simulink model "computer_detect_trafficlight"  (R2016b)
settings: Solver=VariableStepAuto  StartTime=0.0  StopTime=inf  RelTol=1e-3
values from neighbouring files (symbols this model uses):
  h_max_r = hmax(size(hmax,2))    [com_getColor_red.m]    (also in computer_getColor_red.m; computer_getColor_red_video.m)
  h_min_r = hmin(size(hmin,2))    [com_getColor_red.m]    (also in computer_getColor_red.m; computer_getColor_red_video.m)
  s_max_r = smax(size(smax,2))    [com_getColor_red.m]    (also in computer_getColor_red.m; computer_getColor_red_video.m)
  s_min_r = smin(size(smin,2))    [com_getColor_red.m]    (also in computer_getColor_red.m; computer_getColor_red_video.m)
  v_max_r = vmax(size(vmax,2))    [com_getColor_red.m]    (also in computer_getColor_red.m; computer_getColor_red_video.m)
  v_min_r = vmin(size(vmin,2))    [com_getColor_red.m]    (also in computer_getColor_red.m; computer_getColor_red_video.m)
undefined symbols (not defined in the file or in its folder): gray, Rec, SDTV, strel
libraries: dspnetwork x15, visionconversions x5, visionmorphops x2, visiontextngfix x1, xpcrtudplib x1
settings Model: Creator=zeabus  LastModifiedBy=zeabus

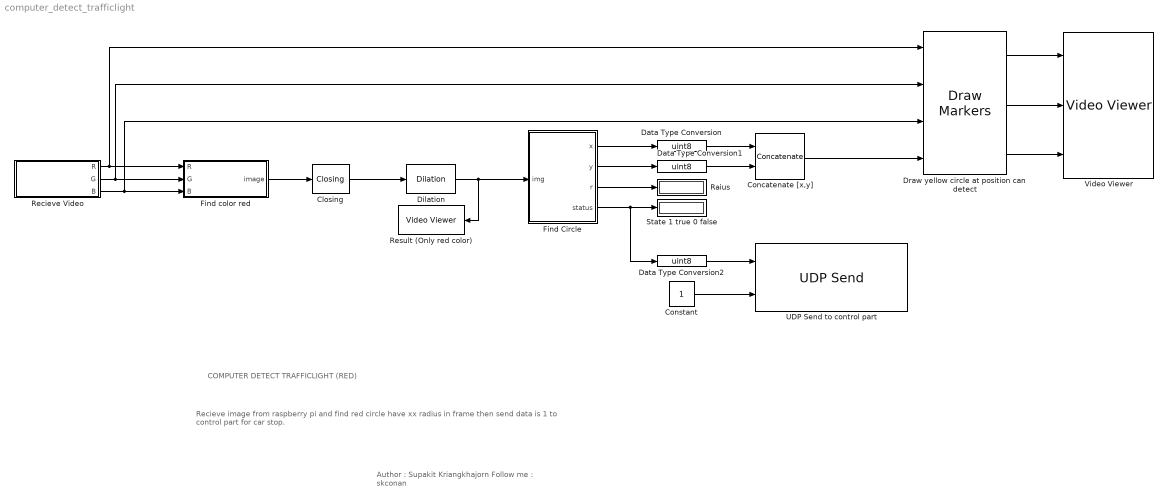
== system computer_detect_trafficlight ==
  note: Recieve image from raspberry pi and find red circle have xx radius in frame then send data is 1 to control part for car stop.
  note: Author : Supakit Kriangkhajorn
      | Follow me : skconan
  note: COMPUTER DETECT TRAFFICLIGHT (RED)
  Closing : visionmorphops/Closing  nhoodsrc=Specify via dialog  strel=strel('line', 10, 40)
  Concatenate [x,y] : Concatenate  Mode=Multidimensional array
  Constant : Constant
  Data Type Conversion : DataTypeConversion  OutDataTypeStr=uint8
  Data Type Conversion1 : DataTypeConversion  OutDataTypeStr=uint8
  Data Type Conversion2 : DataTypeConversion  OutDataTypeStr=uint8
  Dilation : visionmorphops/Dilation  nhoodsrc=Specify via dialog  strel=[35 35 35; 35 35 35; 35 35 35;]
  Draw yellow circle at position can detect : visiontextngfix/Draw Markers  shape=Circle  size=20  fill=on  fillClrSource=Specify via dialog  display=User-specified value  intensity=200  color=[255 255 0]  opacity=0.6  viewport=Entire image  antialiasing=off  inType=Obsolete  imagePorts=Separate color signals  prodOutputMode=Binary point scaling  prodOutputWordLength=32  prodOutputFracLength=14  memoryMode=Specify word length  memoryWordLength=16  memoryFracLength=14  roundingMode=Floor  overflowMode=off
  Find Circle : MATLAB Function  TreatAsAtomicUnit=on
  Find color red : Subsystem
  Raius : Display
  Recieve Video : Subsystem
  Result (Only red color) : VideoViewer  colormapValue=gray(256)  FigPos=[160 608 544 384]
  "State 1 true 0 false " : Display
  "UDP Send to control part " : xpcrtudplib/UDP Send  ipAddressVal=Use host-target connection  localPort=25001  toAddress=192.168.1.118  toPort=20002  sampleTime=0.01
  Video Viewer : VideoViewer  imagePorts=separate color signals  FigPos=[1248 854 490 363]
  wires:
  Draw yellow circle at position can detect/1 -> Video Viewer/1
  Draw yellow circle at position can detect/2 -> Video Viewer/2
  Draw yellow circle at position can detect/3 -> Video Viewer/3
  Find Circle/1(x) -> Data Type Conversion/1
  Find Circle/2(y) -> Data Type Conversion1/1
  Concatenate [x,y]/1 -> Draw yellow circle at position can detect/4
  Data Type Conversion/1 -> Concatenate [x,y]/1
  Data Type Conversion1/1 -> Concatenate [x,y]/2
  Find color red/1(image) -> Closing/1
  Dilation/1 -> Result (Only red color)/1, Find Circle/1(img)
  Find Circle/3(r) -> Raius/1
  Closing/1 -> Dilation/1
  Recieve Video/1(R) -> Draw yellow circle at position can detect/1, Find color red/1(R)
  Recieve Video/2(G) -> Draw yellow circle at position can detect/2, Find color red/2(G)
  Recieve Video/3(B) -> Draw yellow circle at position can detect/3, Find color red/3(B)
  Find Circle/4(status) -> Data Type Conversion2/1, "State 1 true 0 false "/1
  Constant/1 -> "UDP Send to control part "/2
  Data Type Conversion2/1 -> "UDP Send to control part "/1

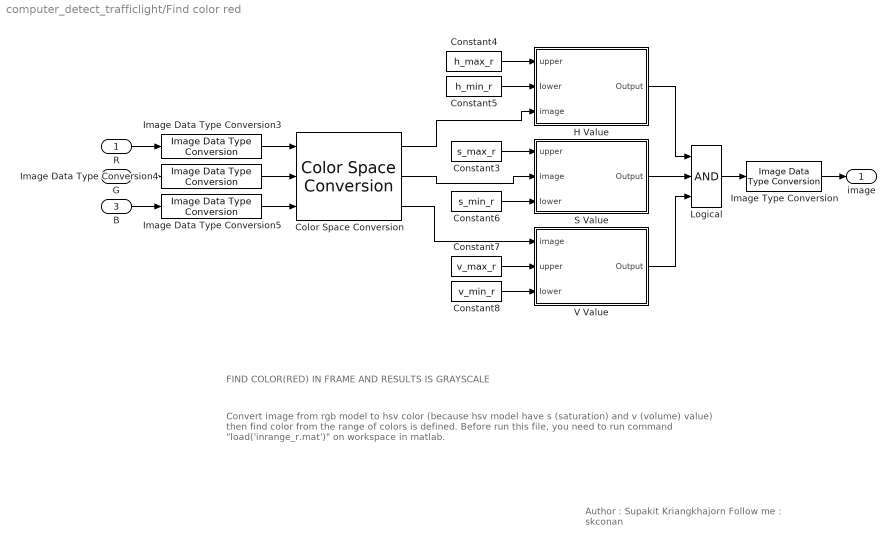
== system computer_detect_trafficlight/Find color red ==
  note: Convert image from rgb model to hsv color (because hsv model have s (saturation) and
      | v (volume) value) then find color from the range of colors is defined.
      |
      | Before run this file, you need to run command "load('inrange_r.mat')" on workspace in matlab.
  note: Author : Supakit Kriangkhajorn
      | Follow me : skconan
  note: FIND COLOR(RED) IN FRAME AND RESULTS IS GRAYSCALE
  R : Inport
  G : Inport  Port=2
  B : Inport  Port=3
  Color Space Conversion : visionconversions/Color Space  Conversion  conversion=Obsolete  conversionActive=R'G'B' to HSV  wp_str=D65  rec=Rec. 601 (SDTV)  sys=1125/60/2:1  imagePorts=Separate color signals
  Constant3 : Constant  Value=s_max_r
  Constant4 : Constant  Value=h_max_r
  Constant5 : Constant  Value=h_min_r
  Constant6 : Constant  Value=s_min_r
  Constant7 : Constant  Value=v_max_r
  Constant8 : Constant  Value=v_min_r
  H Value : Subsystem
  Image Data Type Conversion3 : visionconversions/Image Data Type Conversion  outDT=single  isSigned=on  wordLen=16  numFracBits=0
  Image Data Type Conversion4 : visionconversions/Image Data Type Conversion  outDT=single  isSigned=on  wordLen=16  numFracBits=0
  Image Data Type Conversion5 : visionconversions/Image Data Type Conversion  outDT=single  isSigned=on  wordLen=16  numFracBits=0
  Image Type Conversion : visionconversions/Image Data Type Conversion  outDT=uint8  isSigned=on  wordLen=16  numFracBits=0
  Logical : Logic  Inputs=3  AllPortsSameDT=off  OutDataTypeStr=boolean
  S Value : Subsystem
  V Value : Subsystem
  image : Outport
  wires:
  Color Space Conversion/1 -> H Value/3(image)
  Constant5/1 -> H Value/2(Iower)
  Color Space Conversion/2 -> S Value/2(image)
  Constant3/1 -> S Value/1(upper)
  Constant6/1 -> S Value/3(Iower)
  Color Space Conversion/3 -> V Value/1(image)
  Constant7/1 -> V Value/2(upper)
  Constant8/1 -> V Value/3(Iower)
  H Value/1(Output) -> Logical/1
  S Value/1(Output) -> Logical/2
  V Value/1(Output) -> Logical/3
  Image Data Type Conversion3/1 -> Color Space Conversion/1
  Image Data Type Conversion4/1 -> Color Space Conversion/2
  Image Data Type Conversion5/1 -> Color Space Conversion/3
  Logical/1 -> Image Type Conversion/1
  R/1 -> Image Data Type Conversion3/1
  G/1 -> Image Data Type Conversion4/1
  B/1 -> Image Data Type Conversion5/1
  Constant4/1 -> H Value/1(upper)
  Image Type Conversion/1 -> image/1

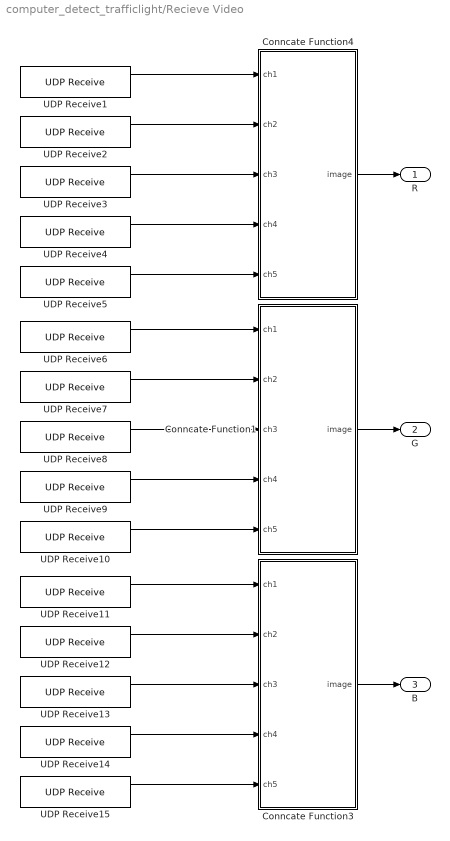
== system computer_detect_trafficlight/Recieve Video ==
  Conncate Function1 : MATLAB Function  TreatAsAtomicUnit=on
  Conncate Function3 : MATLAB Function  TreatAsAtomicUnit=on
  Conncate Function4 : MATLAB Function  TreatAsAtomicUnit=on
  UDP Receive1 : dspnetwork/UDP Receive  localURL='0.0.0.0'  localPort=30000  remoteURL='192.168.1.118'  remotePort=-1  recvBufferSize=15360  dims=15360  signalDatatype=uint8  isVarSize=off  showBlockingTime=on  blockingTime=0  sampletime=1/30  blockPlatform=HOST
  UDP Receive10 : dspnetwork/UDP Receive  localURL='0.0.0.0'  localPort=30009  remoteURL='192.168.1.118'  remotePort=-1  recvBufferSize=15360  dims=15360  signalDatatype=uint8  isVarSize=off  showBlockingTime=on  blockingTime=0  sampletime=1/30  blockPlatform=HOST
  UDP Receive11 : dspnetwork/UDP Receive  localURL='0.0.0.0'  localPort=30010  remoteURL='192.168.1.118'  remotePort=-1  recvBufferSize=15360  dims=15360  signalDatatype=uint8  isVarSize=off  showBlockingTime=on  blockingTime=0  sampletime=1/30  blockPlatform=HOST
  UDP Receive12 : dspnetwork/UDP Receive  localURL='0.0.0.0'  localPort=30011  remoteURL='192.168.1.118'  remotePort=-1  recvBufferSize=15360  dims=15360  signalDatatype=uint8  isVarSize=off  showBlockingTime=on  blockingTime=0  sampletime=1/30  blockPlatform=HOST
  UDP Receive13 : dspnetwork/UDP Receive  localURL='0.0.0.0'  localPort=30012  remoteURL='192.168.1.118'  remotePort=-1  recvBufferSize=15360  dims=15360  signalDatatype=uint8  isVarSize=off  showBlockingTime=on  blockingTime=0  sampletime=1/30  blockPlatform=HOST
  UDP Receive14 : dspnetwork/UDP Receive  localURL='0.0.0.0'  localPort=30013  remoteURL='192.168.1.118'  remotePort=-1  recvBufferSize=15360  dims=15360  signalDatatype=uint8  isVarSize=off  showBlockingTime=on  blockingTime=0  sampletime=1/30  blockPlatform=HOST
  UDP Receive15 : dspnetwork/UDP Receive  localURL='0.0.0.0'  localPort=30014  remoteURL='192.168.1.118'  remotePort=-1  recvBufferSize=15360  dims=15360  signalDatatype=uint8  isVarSize=off  showBlockingTime=on  blockingTime=0  sampletime=1/30  blockPlatform=HOST
  UDP Receive2 : dspnetwork/UDP Receive  localURL='0.0.0.0'  localPort=30001  remoteURL='192.168.1.118'  remotePort=-1  recvBufferSize=15360  dims=15360  signalDatatype=uint8  isVarSize=off  showBlockingTime=on  blockingTime=0  sampletime=1/30  blockPlatform=HOST
  UDP Receive3 : dspnetwork/UDP Receive  localURL='0.0.0.0'  localPort=30002  remoteURL='192.168.1.118'  remotePort=-1  recvBufferSize=15360  dims=15360  signalDatatype=uint8  isVarSize=off  showBlockingTime=on  blockingTime=0  sampletime=1/30  blockPlatform=HOST
  UDP Receive4 : dspnetwork/UDP Receive  localURL='0.0.0.0'  localPort=30003  remoteURL='192.168.1.118'  remotePort=-1  recvBufferSize=15360  dims=15360  signalDatatype=uint8  isVarSize=off  showBlockingTime=on  blockingTime=0  sampletime=1/30  blockPlatform=HOST
  UDP Receive5 : dspnetwork/UDP Receive  localURL='0.0.0.0'  localPort=30004  remoteURL='192.168.1.118'  remotePort=-1  recvBufferSize=15360  dims=15360  signalDatatype=uint8  isVarSize=off  showBlockingTime=on  blockingTime=0  sampletime=1/30  blockPlatform=HOST
  UDP Receive6 : dspnetwork/UDP Receive  localURL='0.0.0.0'  localPort=30005  remoteURL='192.168.1.118'  remotePort=-1  recvBufferSize=15360  dims=15360  signalDatatype=uint8  isVarSize=off  showBlockingTime=on  blockingTime=0  sampletime=1/30  blockPlatform=HOST
  UDP Receive7 : dspnetwork/UDP Receive  localURL='0.0.0.0'  localPort=30006  remoteURL='192.168.1.118'  remotePort=-1  recvBufferSize=15360  dims=15360  signalDatatype=uint8  isVarSize=off  showBlockingTime=on  blockingTime=0  sampletime=1/30  blockPlatform=HOST
  UDP Receive8 : dspnetwork/UDP Receive  localURL='0.0.0.0'  localPort=30007  remoteURL='192.168.1.118'  remotePort=-1  recvBufferSize=15360  dims=15360  signalDatatype=uint8  isVarSize=off  showBlockingTime=on  blockingTime=0  sampletime=1/30  blockPlatform=HOST
  UDP Receive9 : dspnetwork/UDP Receive  localURL='0.0.0.0'  localPort=30008  remoteURL='192.168.1.118'  remotePort=-1  recvBufferSize=15360  dims=15360  signalDatatype=uint8  isVarSize=off  showBlockingTime=on  blockingTime=0  sampletime=1/30  blockPlatform=HOST
  R : Outport
  G : Outport  Port=2
  B : Outport  Port=3
  wires:
  UDP Receive4/1 -> Conncate Function4/4(ch4)
  UDP Receive5/1 -> Conncate Function4/5(ch5)
  UDP Receive3/1 -> Conncate Function4/3(ch3)
  UDP Receive2/1 -> Conncate Function4/2(ch2)
  UDP Receive1/1 -> Conncate Function4/1(ch1)
  UDP Receive9/1 -> Conncate Function1/4(ch4)
  UDP Receive10/1 -> Conncate Function1/5(ch5)
  UDP Receive8/1 -> Conncate Function1/3(ch3)
  UDP Receive7/1 -> Conncate Function1/2(ch2)
  UDP Receive6/1 -> Conncate Function1/1(ch1)
  UDP Receive14/1 -> Conncate Function3/4(ch4)
  UDP Receive15/1 -> Conncate Function3/5(ch5)
  UDP Receive13/1 -> Conncate Function3/3(ch3)
  UDP Receive12/1 -> Conncate Function3/2(ch2)
  UDP Receive11/1 -> Conncate Function3/1(ch1)
  Conncate Function4/1(image) -> R/1
  Conncate Function1/1(image) -> G/1
  Conncate Function3/1(image) -> B/1

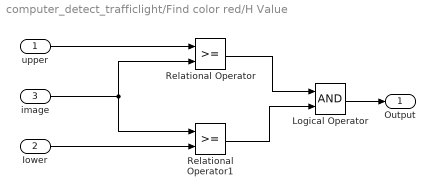
== system computer_detect_trafficlight/Find color red/H Value ==
  upper : Inport
  Iower : Inport  Port=2
  image : Inport  Port=3
  Logical Operator : Logic  AllPortsSameDT=off  OutDataTypeStr=boolean
  Relational Operator : RelationalOperator  OutDataTypeStr=boolean  RndMeth=Simplest
  Relational Operator1 : RelationalOperator  OutDataTypeStr=boolean  RndMeth=Simplest
  Output : Outport
  wires:
  upper/1 -> Relational Operator/1
  Iower/1 -> Relational Operator1/2
  image/1 -> Relational Operator/2, Relational Operator1/1
  Relational Operator/1 -> Logical Operator/1
  Relational Operator1/1 -> Logical Operator/2
  Logical Operator/1 -> Output/1

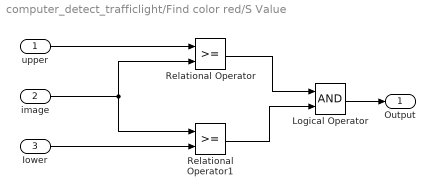
== system computer_detect_trafficlight/Find color red/S Value ==
  upper : Inport
  image : Inport  Port=2
  Iower : Inport  Port=3
  Logical Operator : Logic  AllPortsSameDT=off  OutDataTypeStr=boolean
  Relational Operator : RelationalOperator  OutDataTypeStr=boolean  RndMeth=Simplest
  Relational Operator1 : RelationalOperator  OutDataTypeStr=boolean  RndMeth=Simplest
  Output : Outport
  wires:
  upper/1 -> Relational Operator/1
  Iower/1 -> Relational Operator1/2
  image/1 -> Relational Operator/2, Relational Operator1/1
  Relational Operator/1 -> Logical Operator/1
  Relational Operator1/1 -> Logical Operator/2
  Logical Operator/1 -> Output/1

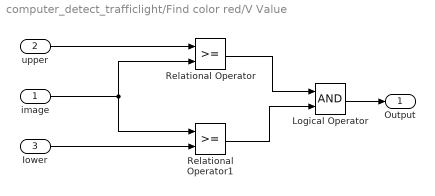
== system computer_detect_trafficlight/Find color red/V Value ==
  image : Inport
  upper : Inport  Port=2
  Iower : Inport  Port=3
  Logical Operator : Logic  AllPortsSameDT=off  OutDataTypeStr=boolean
  Relational Operator : RelationalOperator  OutDataTypeStr=boolean  RndMeth=Simplest
  Relational Operator1 : RelationalOperator  OutDataTypeStr=boolean  RndMeth=Simplest
  Output : Outport
  wires:
  upper/1 -> Relational Operator/1
  Iower/1 -> Relational Operator1/2
  image/1 -> Relational Operator/2, Relational Operator1/1
  Relational Operator/1 -> Logical Operator/1
  Relational Operator1/1 -> Logical Operator/2
  Logical Operator/1 -> Output/1

== matlab function computer_detect_trafficlight/Recieve Video/Conncate Function1 ==
  data: ch1 input; ch2 input; ch3 input; ch4 input; ch5 input uint8; image output
function image  = concatenation(ch1,ch2,ch3,ch4,ch5)
maxcol = 48;
height = 320;
width = 240;
ch1 = reshape(ch1,height,maxcol);
ch2 = reshape(ch2,height,maxcol);
ch3 = reshape(ch3,height,maxcol);
ch4 = reshape(ch4,height,maxcol);
ch5 = reshape(ch5,height,maxcol);
image = [ch1,ch2,ch3,ch4,ch5];
image = reshape(image,height,width);

== matlab function computer_detect_trafficlight/Recieve Video/Conncate Function3 ==
  data: ch1 input; ch2 input; ch3 input; ch4 input; ch5 input uint8; image output
function image  = concatenation(ch1,ch2,ch3,ch4,ch5)
maxcol = 48;
height = 320;
width = 240;
ch1 = reshape(ch1,height,maxcol);
ch2 = reshape(ch2,height,maxcol);
ch3 = reshape(ch3,height,maxcol);
ch4 = reshape(ch4,height,maxcol);
ch5 = reshape(ch5,height,maxcol);
image = [ch1,ch2,ch3,ch4,ch5];
image = reshape(image,height,width);

== matlab function computer_detect_trafficlight/Find Circle ==
  data: img input; x output; y output; r output; status output
% Author : Supakit Kriangkhajorn,'Sensitivity',0.7
% Follow me : skconan

function [x,y,r,status]= findcircle(img)
    coder.extrinsic('imfindcircles'); 
    coder.extrinsic('isempty');
    coder.extrinsic('sortrows');
    coder.extrinsic('size');
    coder.extrinsic('graythresh');
 
    x = 0;
    y = 0;
    r = 0;
    cols = 0;
    status = 0;
    centerMax = [0,0];
 
    [centers, radius, metric] = imfindcircles(img,[17 30],...
                                            'Sensitivity',0.95,...
                                            'Method','twostage',...
                                            'ObjectPolarity','bright');
    circles = [centers, radius, metric];
    check_empty = ~isempty(circles);
    if check_empty 
        status = 1;
        circles = sortrows(circles,3);
        [rows,cols] = size(circles);
        centerMax = circles(rows,1:2);
        r = circles(rows,3);
    end
         
x = round(centerMax(1));
y = round(centerMax(2));

== matlab function computer_detect_trafficlight/Recieve Video/Conncate Function4 ==
  data: ch1 input; ch2 input; ch3 input; ch4 input; ch5 input uint8; image output
function image  = concatenation(ch1,ch2,ch3,ch4,ch5)
maxcol = 48;
height = 320;
width = 240;
ch1 = reshape(ch1,height,maxcol);
ch2 = reshape(ch2,height,maxcol);
ch3 = reshape(ch3,height,maxcol);
ch4 = reshape(ch4,height,maxcol);
ch5 = reshape(ch5,height,maxcol);
image = [ch1,ch2,ch3,ch4,ch5];
image = reshape(image,height,width);
